simulink model "sixpistolets"  (R2017b)
settings: Solver=VariableStepAuto  StartTime=0.0  StopTime=Tsim  RelTol=1e-3
values from neighbouring files (symbols this model uses):
  f1 = 85000    [sixpistolets_script.m]
  f2 = 90000    [sixpistolets_script.m]
  f3 = 94986.6    [sixpistolets_script.m]
  f4 = 100000    [sixpistolets_script.m]
  f5 = 115015.9    [sixpistolets_script.m]
  f6 = 120000    [sixpistolets_script.m]
  Te = T/M    (= 0.03125)    [Script.m]    (also in sixpistolets_script.m = 3.125e-06)
settings Model: Creator=lchauvet  LastModifiedBy=lchauvet

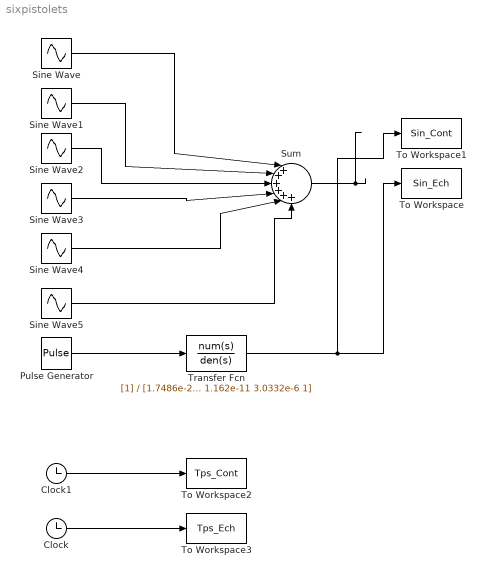
== system sixpistolets ==
  Clock : Clock
  Clock1 : Clock
  Pulse Generator : DiscretePulseGenerator  PulseType=Time based  Period=1/f1  PulseWidth=50
  Sine Wave : Sin  Frequency=2*pi*f1  SampleTime=0
  Sine Wave1 : Sin  Frequency=2*pi*f2  SampleTime=0
  Sine Wave2 : Sin  Frequency=2*pi*f3  SampleTime=0
  Sine Wave3 : Sin  Frequency=2*pi*f4  SampleTime=0
  Sine Wave4 : Sin  Frequency=2*pi*f5  SampleTime=0
  Sine Wave5 : Sin  Frequency=2*pi*f6  SampleTime=0
  Sum : Sum  Inputs=|++++++
  To Workspace : ToWorkspace  VariableName=Sin_Ech  SampleTime=Te
      settings: MaxDataPoints=M
  To Workspace1 : ToWorkspace  VariableName=Sin_Cont  SampleTime=Te/100
      settings: MaxDataPoints=100*M
  To Workspace2 : ToWorkspace  VariableName=Tps_Cont  SampleTime=Te/100
      settings: MaxDataPoints=100*M
  To Workspace3 : ToWorkspace  VariableName=Tps_Ech  SampleTime=Te
      settings: MaxDataPoints=M
  Transfer Fcn : TransferFcn  Denominator=[1.7486e-23 7.6663e-18 1.162e-11 3.0332e-6 1]
  wires:
  Clock1/1 -> To Workspace2/1
  Clock/1 -> To Workspace3/1
  Sine Wave/1 -> Sum/1
  Sine Wave1/1 -> Sum/2
  Sine Wave3/1 -> Sum/4
  Sine Wave4/1 -> Sum/5
  Sine Wave5/1 -> Sum/6
  Sine Wave2/1 -> Sum/3
  Sum/1 -> ?
  Pulse Generator/1 -> Transfer Fcn/1
  Transfer Fcn/1 -> To Workspace1/1, To Workspace/1
